simulink model "pendpid_cntr"  (Simulink 7.1)
settings: Solver=ode3  StartTime=0.0  StopTime=0.3  FixedStep=1e-4  RelTol=1e-3  AbsTol=1e-6
settings Model: Creator=Pogorelov  LastModifiedBy=kovalev
settings DataIOCC: LimitDataPoints=off
settings OptimizationCC: BlockReduction=off  BooleanDataType=off
settings DebuggingCC: SaveWithParameterizedLinksMsg=none  SignalResolutionControl=TryResolveAllWithWarning  SolverPrmCheckMsg=none  MultiTaskDSMMsg=warning  MultiTaskCondExecSysMsg=none  StrictBusMsg=None
settings HardwareCC: TargetUnknown=on
settings RTWCC: GenerateMakefile=off  TemplateMakefile=grt_vc.tmf  IncludeERTFirstTime=on
settings GRTTargetCC: ExtModeMexFile=noextcomm

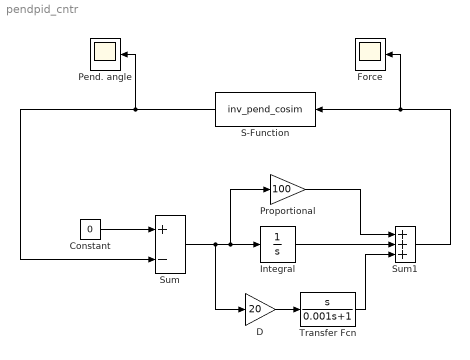
== system pendpid_cntr ==
  Constant : Constant  Value=0
  D : Gain  Gain=20  SaturateOnIntegerOverflow=on  OutDataTypeStr=Inherit: Same as input  ParamDataTypeStr=Inherit: Same as input
  Force : Scope
      settings: YMin=-7000  YMax=1000  MaxDataPoints=50000
  Integral : TransferFcn  Denominator=[1 0]
  Pend. angle : Scope
      settings: TimeRange=0.3  YMin=-0.1  YMax=0.3  MaxDataPoints=500000
  Proportional : Gain  Gain=100  SaturateOnIntegerOverflow=on  OutDataTypeStr=Inherit: Same as input  ParamDataTypeStr=Inherit: Same as input
  S-Function : S-Function  Orientation=left  FunctionName=inv_pend_cosim  EnableBusSupport=off
  Sum : Sum  Inputs=+-  SaturateOnIntegerOverflow=on  InputSameDT=on  OutDataTypeStr=Inherit: Same as first input
  Sum1 : Sum  Inputs=+++  SaturateOnIntegerOverflow=on  InputSameDT=on  OutDataTypeStr=Inherit: Same as first input
  Transfer Fcn : TransferFcn  Numerator=[1 0]  Denominator=[0.001 1]
  wires:
  Constant/1 -> Sum/1
  D/1 -> Transfer Fcn/1
  Sum/1 -> D/1, Proportional/1, Integral/1
  Transfer Fcn/1 -> Sum1/3
  Integral/1 -> Sum1/2
  Proportional/1 -> Sum1/1
  Sum1/1 -> S-Function/1, Force/1
  S-Function/1 -> Sum/2, Pend. angle/1
